simulink model "baleka_simscape"  (R2024b)
settings: Solver=VariableStepAuto  StartTime=0.0  StopTime=1  RelTol=1e-3
InitFcn:
  | VLcmdsignal = struct( ...
  |     'r_des', 0.4, ...
  |     'dr_des', 0, ...
  |     'th_des', -pi/2, ...
  |     'dth_des', 0, ...
  |     'KPr', 500, ...
  |     'KDr', 10, ...
  |     'KPth', 50, ...
  |     'KDth', 5, ...
  |     'Fff', 0, ...
  |     'Tff', 0);
libraries: aru_toolbox x3
settings Model: DataDictionary=Library_dictionary.sldd  Creator=claro  LastModifiedBy=claro

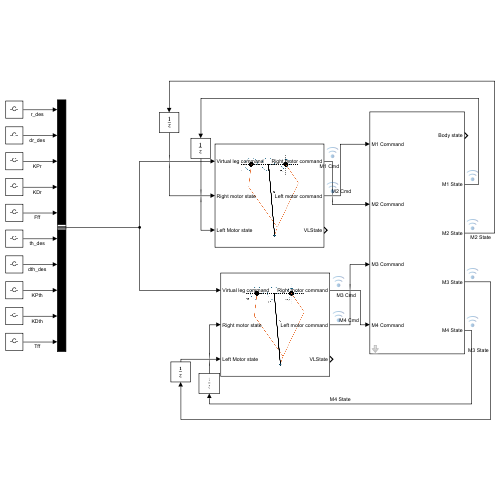
[thumbnail: Simulink's stored preview of the top-level diagram]
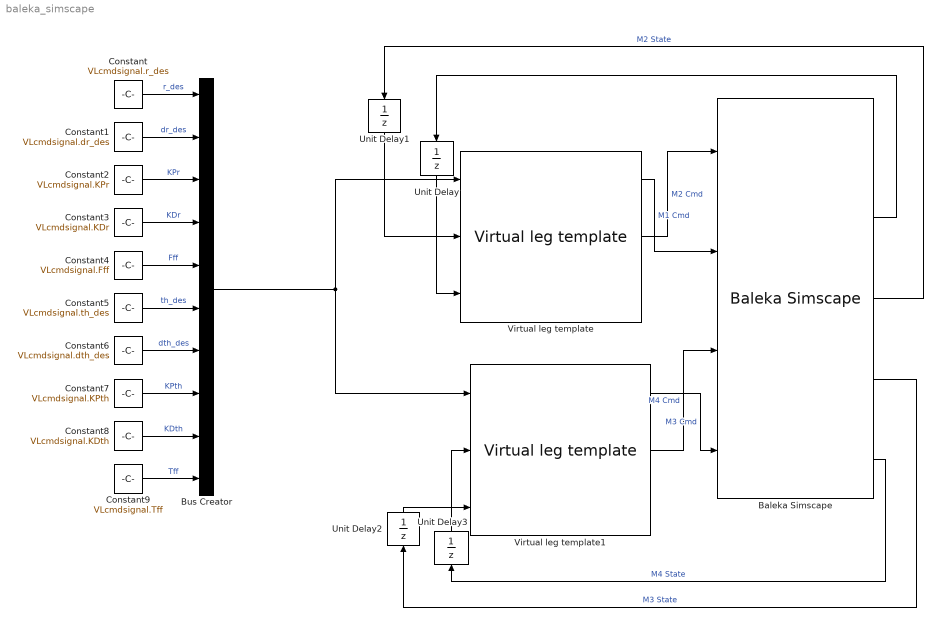
== system baleka_simscape ==
  Baleka Simscape : aru_toolbox/Baleka 2.5/Baleka Simscape  communication_rate=1000  GravityBool=on  mu_s=1  mu_k=0.9  foot_k=1e5  foot_d=1e4  y_start=0.5  StartingMode=Links horizontal  LOffset=3*pi/2  ROffset=-pi/2
      settings: SourceProductName=ARU Toolbox
  Bus Creator : BusCreator  Inputs=10  OutDataTypeStr=Bus: VLcmd
  Constant : Constant  Value=VLcmdsignal.r_des
  Constant1 : Constant  Value=VLcmdsignal.dr_des
  Constant2 : Constant  Value=VLcmdsignal.KPr
  Constant3 : Constant  Value=VLcmdsignal.KDr
  Constant4 : Constant  Value=VLcmdsignal.Fff
  Constant5 : Constant  Value=VLcmdsignal.th_des
  Constant6 : Constant  Value=VLcmdsignal.dth_des
  Constant7 : Constant  Value=VLcmdsignal.KPth
  Constant8 : Constant  Value=VLcmdsignal.KDth
  Constant9 : Constant  Value=VLcmdsignal.Tff
  Unit Delay{,1..3} (4 alike) : UnitDelay  SampleTime=-1  HasFrameUpgradeWarning=on
  Virtual leg template : aru_toolbox/Baleka 2.5/Virtual leg template  SystemSampleTime=-1  VariantActivationTime=update diagram  AllowFlexibleInterface=on  Latency=0  AutoFrameSizeCalculation=off
      settings: SourceProductName=ARU Toolbox
  Virtual leg template1 : aru_toolbox/Baleka 2.5/Virtual leg template  SystemSampleTime=-1  VariantActivationTime=update diagram  AllowFlexibleInterface=on  Latency=0  AutoFrameSizeCalculation=off
      settings: SourceProductName=ARU Toolbox
  wires:
  Virtual leg template/2 -> Baleka Simscape/1  "M2 Cmd"
  Virtual leg template/1 -> Baleka Simscape/2  "M1 Cmd"
  Virtual leg template1/1 -> Baleka Simscape/4  "M3 Cmd"
  Virtual leg template1/2 -> Baleka Simscape/3  "M4 Cmd"
  Baleka Simscape/2 -> Unit Delay/1
  Baleka Simscape/3 -> Unit Delay1/1  "M2 State"
  Baleka Simscape/4 -> Unit Delay2/1  "M3 State"
  Baleka Simscape/5 -> Unit Delay3/1  "M4 State"
  Bus Creator/1 -> Virtual leg template/1, Virtual leg template1/1
  Constant/1 -> Bus Creator/1  "r_des"
  Constant1/1 -> Bus Creator/2  "dr_des"
  Constant2/1 -> Bus Creator/3  "KPr"
  Constant3/1 -> Bus Creator/4  "KDr"
  Constant4/1 -> Bus Creator/5  "Fff"
  Constant5/1 -> Bus Creator/6  "th_des"
  Constant6/1 -> Bus Creator/7  "dth_des"
  Constant7/1 -> Bus Creator/8  "KPth"
  Constant8/1 -> Bus Creator/9  "KDth"
  Constant9/1 -> Bus Creator/10  "Tff"
  Unit Delay/1 -> Virtual leg template/3
  Unit Delay1/1 -> Virtual leg template/2
  Unit Delay2/1 -> Virtual leg template1/3
  Unit Delay3/1 -> Virtual leg template1/2
